simulink model "lab3_zq"  (R2013b)
settings: Solver=ode45  SolverMode=SingleTasking  StartTime=0.0  StopTime=t_max  MaxStep=0.1  RelTol=1e-3
undefined symbols (not defined in the file): Lo, Lrz, Mo, Mrz, T, t0, y0
settings Model: CovMetricSettings=dwe  CovHtmlReporting=off  covSaveCumulativeToWorkspaceVar=off  CovSaveSingleToWorkspaceVar=off  CovExternalEMLEnable=on  Creator=lev  LastModifiedBy=lev
settings DataIOCC: LimitDataPoints=off  SaveFormat=StructureWithTime
settings DebuggingCC: UnderspecifiedInitializationDetection=Simplified  MergeDetectMultiDrivingBlocksExec=error  SolverPrmCheckMsg=none  FrameProcessingCompatibilityMsg=error  SFUnexpectedBacktrackingDiag=error  SFNoUnconditionalDefaultTransitionDiag=error
settings HardwareCC: ProdBitPerPointer=64  ProdLargestAtomicFloat=Float  ProdIntDivRoundTo=Zero  ProdEndianess=LittleEndian  ProdHWDeviceType=Specified
settings ModelReferenceCC: PropagateSignalLabelsOutOfModel=on
settings SFSimCC: SimUseLocalCustomCode=on
settings RTWCC: RTWUseLocalCustomCode=on
settings GRTTargetCC: CodeReplacementLibrary=C99 (ISO)  GeneratePreprocessorConditionals=Use local settings

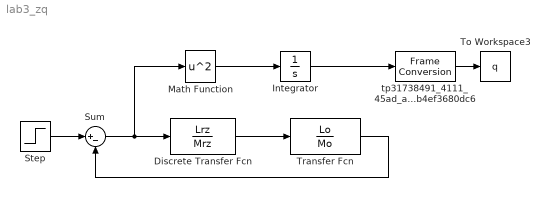
== system lab3_zq ==
  Discrete Transfer Fcn : DiscreteTransferFcn  Numerator=Lrz  Denominator=Mrz  SampleTime=T
  Integrator : Integrator
  Math Function : Math  Operator=square  SaturateOnIntegerOverflow=on
  Step : Step  Time=t0  After=y0  SampleTime=0
  Sum : Sum  Inputs=|+-
  To Workspace3 : ToWorkspace  VariableName=q  SampleTime=-1
      settings: MaxDataPoints=1
  Transfer Fcn : TransferFcn  Numerator=Lo  Denominator=Mo
  tp31738491_4111_45ad_a906_eb4ef3680dc6 : FrameConversion  OutFrame=Sample-based
  wires:
  Transfer Fcn/1 -> Sum/2
  Sum/1 -> Discrete Transfer Fcn/1, Math Function/1
  Step/1 -> Sum/1
  Math Function/1 -> Integrator/1
  Discrete Transfer Fcn/1 -> Transfer Fcn/1
  Integrator/1 -> tp31738491_4111_45ad_a906_eb4ef3680dc6/1
  tp31738491_4111_45ad_a906_eb4ef3680dc6/1 -> To Workspace3/1
